simulink subsystem "AOO_mode"  (R2022a)
settings: Solver=VariableStepAuto  StartTime=0.0  StopTime=10.0  RelTol=1e-3
settings Model: Creator=ivanl  LastModifiedBy=ivanl

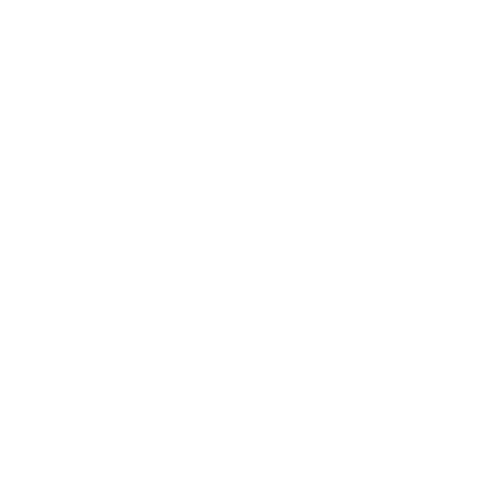
[thumbnail: Simulink's stored preview of the top-level diagram]
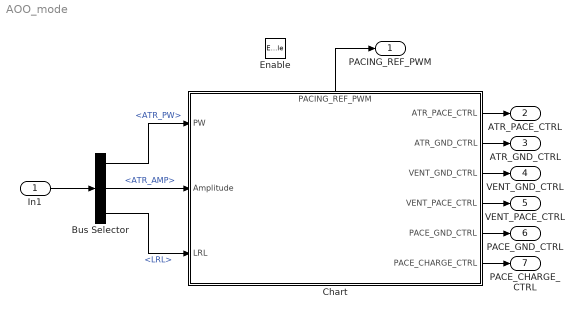
== system AOO_mode ==
  In1 : Inport
  Enable : EnablePort
  Bus Selector : BusSelector  OutputSignals=ATR_PW,ATR_AMP,LRL
  Chart : Stateflow chart  TreatAsAtomicUnit=on
      settings: PortSchema="{\"entries\":[{\"content\":{\"sides\":[{\"content\":{\"connectorIds\":[\"In1\",\"In2\",\"In3\"]},\"type\":\"ConnectorPlacement.EquallySpacedRectSide\",\"uuid\":\"2dca410f-8f43-416b-b245-db6a1c9e2101\"},{\"content\":{\"connectorIds\":[\"Out2\",\"Out1\",\"Out4\",\"Out5\",\"Out6\",\"Out3\"],\"side\":\"RIGHT\"},\"type\":\"ConnectorPlacement.EquallySpacedRectSide\",\"uuid\":\"30508f3d-7d2b-4c80-aa19-382c3c260e83\"},{\"content\":{\"connectorIds\":[\"Out7\"],\"side\":\"TOP\"},\"type\":\"ConnectorPlacement.EquallySpacedRectSide\",\"uuid\":\"0cf054d9-a9d5-4fcc-8b60-c098224d8790\"}]},\"type\":\"ConnectorPlacement.EquallySpacedConnector\",\"uuid\":\"125de75b-c166-48e2-8d91-77ead1c82200\"}],\"packageUris\":[\"http://schema.mathworks.com/mf0/Connector/R2020b\"],\"version\":\"1.0\"}"
  PACING_REF_PWM : Outport
  ATR_PACE_CTRL : Outport  Port=2
  ATR_GND_CTRL : Outport  Port=3
  VENT_GND_CTRL : Outport  Port=4
  VENT_PACE_CTRL : Outport  Port=5
  PACE_GND_CTRL : Outport  Port=6
  PACE_CHARGE_CTRL : Outport  Port=7
  wires:
  Chart/2(ATR_PACE_CTRL) -> ATR_PACE_CTRL/1
  Chart/1(ATR_GND_CTRL) -> ATR_GND_CTRL/1
  Chart/4(VENT_GND_CTRL) -> VENT_GND_CTRL/1
  Chart/5(VENT_PACE_CTRL) -> VENT_PACE_CTRL/1
  Chart/6(PACE_GND_CTRL) -> PACE_GND_CTRL/1
  Chart/3(PACE_CHARGE_CTRL) -> PACE_CHARGE_CTRL/1
  Chart/7(PACING_REF_PWM) -> PACING_REF_PWM/1
  Bus Selector/3 -> Chart/3(LRL)  "<LRL>"
  Bus Selector/1 -> Chart/1(PW)  "<ATR_PW>"
  Bus Selector/2 -> Chart/2(Amplitude)  "<ATR_AMP>"
  In1/1 -> Bus Selector/1

== stateflow chart AOO_mode/Chart ==
  state AOO_Charging_C22
    entry:
    VENT_PACE_CTRL = false;
    ATR_PACE_CTRL = false;
    PACE_CHARGE_CTRL = true;
    PACING_REF_PWM = Amplitude * 20;
    PACE_GND_CTRL= true;
    VENT_GND_CTRL = false;
    ATR_GND_CTRL = true;
  state AOO_Pacing
    entry:
    PACE_CHARGE_CTRL = false;
    PACE_GND_CTRL = true;
    VENT_PACE_CTRL = false;
    VENT_GND_CTRL = false;
    ATR_GND_CTRL = false;
    ATR_PACE_CTRL = true;
  (default) -> AOO_Charging_C22
  AOO_Charging_C22 -> AOO_Pacing : after(((60000/LRL) - PW), msec)
  AOO_Pacing -> AOO_Charging_C22 : after(PW, msec)
  data: ATR_GND_CTRL output boolean; ATR_PACE_CTRL output boolean; PACE_CHARGE_CTRL output boolean; VENT_GND_CTRL output boolean; VENT_PACE_CTRL output boolean; PACE_GND_CTRL output boolean; PW input double; Amplitude input double; LRL input double; PACING_REF_PWM output double
